simulink model "step9_power_8"  (R2025a)
settings: Solver=ode45  StartTime=0.0  StopTime=20  MaxStep=0.01  RelTol=1e-3
undefined symbols (not defined in the file or in its folder): A, B, F, K, R
libraries: SignalEditorBlockLib x1
settings Model: Creator=O M E N  LastModifiedBy=O M E N

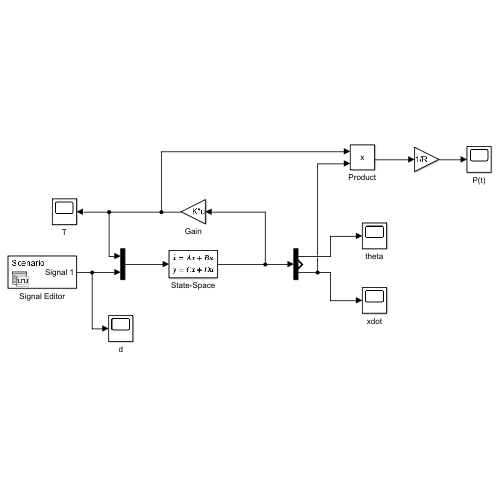
[thumbnail: Simulink's stored preview of the top-level diagram]
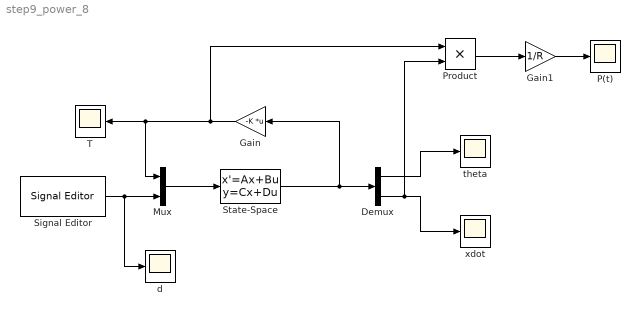
== system step9_power_8 ==
  Demux : Demux  Outputs=3
  Gain : Gain  Gain=-K  Multiplication=Matrix(K*u)
  Gain1 : Gain  Gain=1/R
  Mux : Mux  Inputs=2
  P(t) : Scope
      settings: Title=Mechanical power P(t)  ActiveDisplayYMinimum=-1.471190841214431  ActiveDisplayYMaximum=1.8067955425419178  YLabel="P  (W)"  DataLoggingVariableName=ScopeData4
  Product : Product
  Signal Editor : SignalEditorBlockLib/Signal Editor  FileName=d_trapezoid.mat  ActiveScenario=Scenario  ActiveSignal=Signal 1  IsBus=off  OutputBusObjectStr=Bus: BusObject  SampleTime=0  ZeroCross=off  OutputAfterFinalValue=Setting to zero  Unit=inherit  PreserveSignalName=on  ApplySigPropsToAllScenarios=on  ApplySigPropsToAllSignals=off  SignalPropertySource=Dialog parameters
  State-Space : StateSpace  A=A  B=[B F]  C=eye(3)  D=zeros(3,2)  InitialCondition=[0; 0; 0]
  T : Scope
      settings: Title=Control torque T(t)  ActiveDisplayYMinimum=-6.2475939827700566  ActiveDisplayYMaximum=6.658573334300919  YLabel="T  (N·m)"  DataLoggingVariableName=ScopeData2
  d : Scope
      settings: Title=Disturbance d(t)  ActiveDisplayYMinimum=-0.0012499999999999998  ActiveDisplayYMaximum=0.01125  YLabel="d  (m)"  DataLoggingVariableName=ScopeData3
  theta : Scope
      settings: Title=Tilt angle θ(t)  ActiveDisplayYMinimum=-0.011067084420853352  ActiveDisplayYMaximum=0.0012601577879934294  YLabel="θ  (rad)"
  xdot : Scope
      settings: Title=Vehicle speed ẋ(t)  ActiveDisplayYMinimum=-0.024282492577397681  ActiveDisplayYMaximum=0.14170516443992251  YLabel="ẋ  (m/s)"
  wires:
  Mux/1 -> State-Space/1
  State-Space/1 -> Gain/1, Demux/1
  Gain/1 -> Product/1, T/1, Mux/1
  Signal Editor/1 -> d/1, Mux/2
  Demux/1 -> theta/1
  Demux/3 -> Product/2, xdot/1
  Product/1 -> Gain1/1
  Gain1/1 -> P(t)/1
